simulink model "c2000_model_pil_block"  (R2021b)
settings: Solver=FixedStepDiscrete  StartTime=0.0  StopTime=10  FixedStep=T  RelTol=1e-3
PostLoadFcn:
  | Increment = Simulink.Parameter;
  | Increment.DataType = 'uint8';
  | Increment.CoderInfo.StorageClass = 'SimulinkGlobal';
  | Increment.Value = 1;
  | 
  | SilCounterBus = Simulink.Bus;
  | SilCounterBus.Description = 'This bus contains counter inputs';
  | 
  | e1 = Simulink.BusElement;
  | e1.DataType = 'boolean';
  | e1.Name = 'ticks_to_count';
  | 
  | e2 = Simulink.BusElement;
  | e2.DataType = 'boolean';
  | e2.Name = 'reset';
  | 
  | SilCounterBus.Elements = [e1 e2];
  | clear e1 e2
  | 
  | % Step size
  | T=0.1;
  | 
  | % Input values
  | ticks_to_count.time = (0:100)'*T;
  | ticks_to_count.signals.values = boolean((floor( (0:100)/2)==(0:100)/2)');
  | ticks_to_count.signals.dimensions = 1;
  | 
  | reset.time = (0:100)'*T;
  | reset_values = boolean(zeros(101,1)); reset_values(20)=true;
  | reset.signals.values = reset_values;
  | clear reset_values
  | reset.signals.dimensions = 1;
Description:
  | Processor-in-the-Loop Code Verification
settings Model: FPTRunName=Active  ExtModeTrigDuration=8  Creator=The MathWorks, Inc.  LastModifiedBy=The MathWorks, Inc.
settings SolverCC: AlgebraicLoopSolver=TrustRegion
settings DataIOCC: SaveFormat=StructureWithTime  SaveOutput=off  SaveTime=off  SignalLoggingName=logsOut
settings OptimizationCC: UseDivisionForNetSlopeComputation=UseDivisionForReciprocalsOfIntegersOnly  EnhancedBackFolding=on  BooleansAsBitfields=on  PassReuseOutputArgsAs=Individual arguments  ExpressionDepthLimit=2147483647  StateBitsets=on  DataBitsets=on  NoFixptDivByZeroProtection=on  EfficientFloat2IntCast=on  LifeSpan=1  MaxStackSize=512  SimCompilerOptimization=on  DenormalBehavior=FlushToZero  EfficientTunableParamExpr=on
settings DebuggingCC: ReadBeforeWriteMsg=DisableAll  WriteAfterWriteMsg=DisableAll  WriteAfterReadMsg=DisableAll  UnderspecifiedInitializationDetection=Classic  CheckExecutionContextPreStartOutputMsg=on  FcnCallInpInsideContextMsg=warning  UniqueDataStoreMsg=error  AllowSymbolicDim=off  ModelReferenceSymbolNameMessage=none  StateNameClashWarn=warning  StrictBusMsg=ErrorOnBusTreatedAsVector  SymbolicDimsDataTypeCodeGenerationDiagnostic=none  SFUnexpectedBacktrackingDiag=warning  SFNoUnconditionalDefaultTransitionDiag=warning  SFExecutionAtInitializationDiag=none  SFMachineParentedDataDiag=warning  ArithmeticOperatorsInVariantConditions=warning
settings HardwareCC: ProdBitPerChar=16  ProdBitPerInt=16  ProdBitPerPointer=32  ProdBitPerSizeT=32  ProdBitPerPtrDiffT=32  ProdLargestAtomicInteger=Integer  ProdLargestAtomicFloat=None  ProdWordSize=16  ProdLongLongMode=on  ProdHWDeviceType=Texas Instruments->C2000  TargetHWDeviceType=Generic->32-bit Embedded Processor
settings ModelReferenceCC: CheckModelReferenceTargetMessage=none  PropagateSignalLabelsOutOfModel=off
settings SFSimCC: SimUseLocalCustomCode=off  MATLABDynamicMemAlloc=off
settings RTWCC: Description=Embedded Coder  SystemTargetFile=ert.tlc  HardwareBoard=TI Piccolo F2806x  TemplateMakefile=ert_default_tmf  GenerateReport=on  RTWVerbose=off  RTWUseLocalCustomCode=off  Toolchain=Texas Instruments Code Composer Studio (C2000)  IncludeHyperlinkInReport=on  CodeProfilingSaveOptions=AllData  GenerateTraceInfo=on  GenerateTraceReport=on  GenerateTraceReportSl=on  GenerateTraceReportSf=on  GenerateTraceReportEml=on  GenerateCodeMetricsReport=on
settings CodeAppCC: ForceParamTrailComments=on  IgnoreCustomStorageClasses=off  SimulinkDataObjDesc=on  CustomSymbolStrGlobalVar=rt$N$M  CustomSymbolStrType=$N$M  CustomSymbolStrFcn=$N$M$F  CustomSymbolStrMacro=$N$M  InsertBlockDesc=on  StateflowObjectComments=on  InternalIdentifier=Classic
settings ERTTargetCC: CodeReplacementLibrary=TI C28x  UtilityFuncGeneration=Shared location  MultiwordLength=2048  IncludeMdlTerminateFcn=off  CombineSignalStateStructs=on  SupportNonFinite=off  SupportComplex=off  ExtModeStaticAllocSize=2048  ERTFilePackagingFormat=CompactWithDataFile  ConvertIfToSwitch=off  SuppressUnreachableDefaultCases=off
settings ConfigComp: CovMetricSettings=dw  CovSaveCumulativeToWorkspaceVar=on  CovSaveSingleToWorkspaceVar=on  CovExternalEMLEnable=off  CovSFcnEnable=off

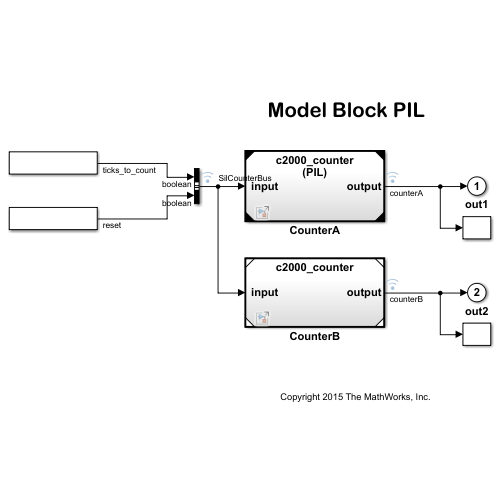
[thumbnail: Simulink's stored preview of the top-level diagram]
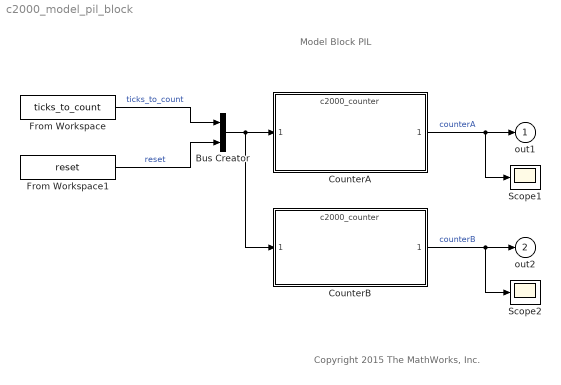
== system c2000_model_pil_block ==
  note: Copyright 2015 The MathWorks, Inc.
  note: Model Block PIL
  Bus Creator : BusCreator  Inputs='ticks_to_count','reset'  OutDataTypeStr=Bus: SilCounterBus  NonVirtualBus=on
  CounterA : ModelReference  ModelNameDialog=c2000_counter  UsingDefaultArgumentValue=0,0  SimulationMode=Processor-in-the-loop (PIL)  ModelReferenceVersion=1.155
  CounterB : ModelReference  ModelNameDialog=c2000_counter  UsingDefaultArgumentValue=0,0  SimulationMode=Normal  ModelReferenceVersion=1.155
  From Workspace : FromWorkspace  VariableName=ticks_to_count  SampleTime=T
  From Workspace1 : FromWorkspace  VariableName=reset  SampleTime=T
  Scope1 : Scope
  Scope2 : Scope
  out1 : Outport  VectorParamsAs1DForOutWhenUnconnected=off
  out2 : Outport  Port=2  VectorParamsAs1DForOutWhenUnconnected=off
  wires:
  CounterA/1 -> Scope1/1, out1/1  "counterA"
  Bus Creator/1 -> CounterA/1, CounterB/1
  From Workspace/1 -> Bus Creator/1  "ticks_to_count"
  From Workspace1/1 -> Bus Creator/2  "reset"
  CounterB/1 -> out2/1, Scope2/1  "counterB"
